simulink model "Inverted_pendulum_simulation"  (R2015a)
settings: Solver=ode45  StartTime=0.0  StopTime=20  RelTol=1e-3
values from neighbouring files (symbols this model uses):
  K = lqr(A,B,Q,R)    [Initialize_model.m]
settings Model: Creator=HP  LastModifiedBy=HP

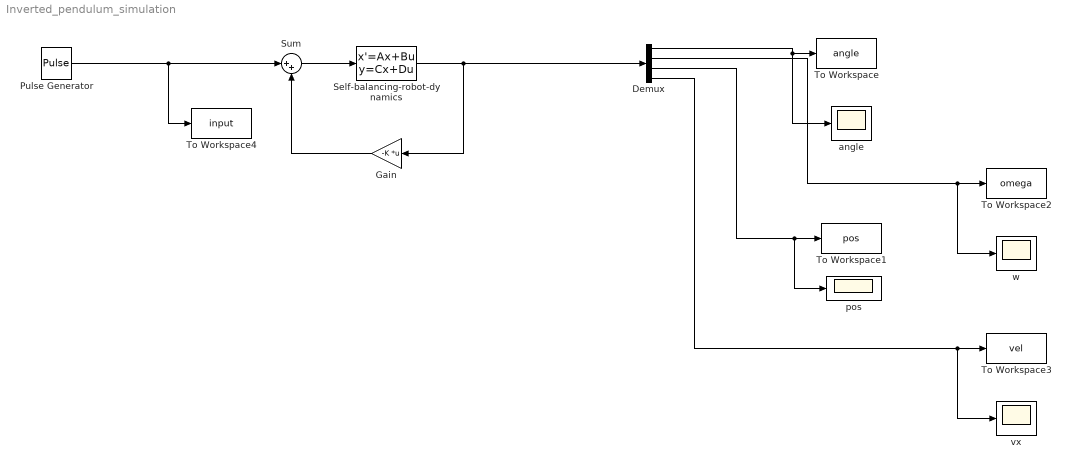
== system Inverted_pendulum_simulation ==
  Demux : Demux
  Gain : Gain  Gain=-K  Multiplication=Matrix(K*u)
  Pulse Generator : DiscretePulseGenerator  PulseType=Time based  Amplitude=5  Period=10  PulseWidth=50
  Self-balancing-robot-dynamics : StateSpace  A=[0,1,0,0; 0,16.33,0,0; 0,0,0,1; 0,130.7,0,0]  B=[0;4.444;0;22.22]  C=[1 0 0 0; 0 1 0 0; 0 0 1 0; 0 0 0 1]  D=[0;0;0;0]  X0=[0 0 0 0]  ContinuousStateAttributes='x'
  Sum : Sum  Inputs=|++
  To Workspace : ToWorkspace  VariableName=angle  SaveFormat=Timeseries  SampleTime=-1
  To Workspace1 : ToWorkspace  VariableName=pos  SaveFormat=Timeseries  SampleTime=-1
  To Workspace2 : ToWorkspace  VariableName=omega  SaveFormat=Timeseries  SampleTime=-1
  To Workspace3 : ToWorkspace  VariableName=vel  SaveFormat=Timeseries  SampleTime=-1
  To Workspace4 : ToWorkspace  VariableName=input  SaveFormat=Timeseries  SampleTime=-1
  angle : Scope
      settings: TickLabels=on  ShowLegends=on  YMin=0  ScrollMode=on
  pos : Scope
      settings: YMin=-4e+17  YMax=4e+17  SaveName=ScopeData3  ScrollMode=on
  vx : Scope
      settings: TickLabels=on  ShowLegends=on  YMin=0  SaveName=ScopeData2  ScrollMode=on
  w : Scope
      settings: TickLabels=on  ShowLegends=on  YMin=0  ScrollMode=on
  wires:
  Self-balancing-robot-dynamics/1 -> Demux/1, Gain/1
  Demux/1 -> angle/1, To Workspace/1
  Demux/3 -> pos/1, To Workspace1/1
  Demux/2 -> To Workspace2/1, w/1
  Demux/4 -> vx/1, To Workspace3/1
  Sum/1 -> Self-balancing-robot-dynamics/1
  Gain/1 -> Sum/2
  Pulse Generator/1 -> To Workspace4/1, Sum/1
